simulink model "TrajectoryGenerator2DOF"  (R2023b)
settings: Solver=FixedStepDiscrete  StartTime=0.0  StopTime=1.538*1.4  FixedStep=0.002  RelTol=1e-3
undefined symbols (not defined in the file or in its folder): M_z, Smoothers, Ts
(part 2 of 3)

== system TrajectoryGenerator2DOF/Trajectory Generator10/M23 ==
  x : Inport
  Discrete FIR Filter1 : DiscreteFir  Coefficients=1/N/Ts*[1 zeros(1,N-1) -1]  InitialStates=Q0  SampleTime=Ts
  Discrete Filter : DiscreteFilter  Numerator=[0 Ts]  Denominator=[1 -1]  InitialStates=Q0  SampleTime=Ts
  y : Outport
  dy : Outport  Port=2
  wires:
  Discrete FIR Filter1/1 -> Discrete Filter/1, dy/1
  x/1 -> Discrete FIR Filter1/1
  Discrete Filter/1 -> y/1

== system TrajectoryGenerator2DOF/Trajectory Generator10/M24 ==
  x : Inport
  Discrete FIR Filter1 : DiscreteFir  Coefficients=1/N/Ts*[1 zeros(1,N-1) -1]  InitialStates=Q0  SampleTime=Ts
  Discrete Filter : DiscreteFilter  Numerator=[0 Ts]  Denominator=[1 -1]  InitialStates=Q0  SampleTime=Ts
  y : Outport
  dy : Outport  Port=2
  wires:
  Discrete FIR Filter1/1 -> Discrete Filter/1, dy/1
  x/1 -> Discrete FIR Filter1/1
  Discrete Filter/1 -> y/1

== system TrajectoryGenerator2DOF/Trajectory Generator10/M33 ==
  x : Inport
  Discrete FIR Filter1 : DiscreteFir  Coefficients=1/N/Ts*[1 zeros(1,N-1) -1]  InitialStates=Q0  SampleTime=Ts
  Discrete Filter : DiscreteFilter  Numerator=[0 Ts]  Denominator=[1 -1]  InitialStates=Q0  SampleTime=Ts
  y : Outport
  dy : Outport  Port=2
  wires:
  Discrete FIR Filter1/1 -> Discrete Filter/1, dy/1
  x/1 -> Discrete FIR Filter1/1
  Discrete Filter/1 -> y/1

== system TrajectoryGenerator2DOF/Trajectory Generator10/M34 ==
  x : Inport
  Discrete FIR Filter1 : DiscreteFir  Coefficients=1/N/Ts*[1 zeros(1,N-1) -1]  InitialStates=Q0  SampleTime=Ts
  Discrete Filter : DiscreteFilter  Numerator=[0 Ts]  Denominator=[1 -1]  InitialStates=Q0  SampleTime=Ts
  y : Outport
  dy : Outport  Port=2
  wires:
  Discrete FIR Filter1/1 -> Discrete Filter/1, dy/1
  x/1 -> Discrete FIR Filter1/1
  Discrete Filter/1 -> y/1

== system TrajectoryGenerator2DOF/Trajectory Generator10/M44 ==
  x : Inport
  Discrete FIR Filter1 : DiscreteFir  Coefficients=1/N/Ts*[1 zeros(1,N-1) -1]  InitialStates=Q0  SampleTime=Ts
  Discrete Filter : DiscreteFilter  Numerator=[0 Ts]  Denominator=[1 -1]  InitialStates=Q0  SampleTime=Ts
  y : Outport
  dy : Outport  Port=2
  wires:
  Discrete FIR Filter1/1 -> Discrete Filter/1, dy/1
  x/1 -> Discrete FIR Filter1/1
  Discrete Filter/1 -> y/1

== system TrajectoryGenerator2DOF/Trajectory Generator11/M11 ==
  x : Inport
  Discrete FIR Filter1 : DiscreteFir  Coefficients=1/N/Ts*[1 zeros(1,N-1) -1]  InitialStates=Q0  SampleTime=Ts
  Discrete Filter : DiscreteFilter  Numerator=[0 Ts]  Denominator=[1 -1]  InitialStates=Q0  SampleTime=Ts
  y : Outport
  dy : Outport  Port=2
  wires:
  Discrete FIR Filter1/1 -> Discrete Filter/1, dy/1
  x/1 -> Discrete FIR Filter1/1
  Discrete Filter/1 -> y/1

== system TrajectoryGenerator2DOF/Trajectory Generator11/M12 ==
  x : Inport
  Discrete FIR Filter1 : DiscreteFir  Coefficients=1/N/Ts*[1 zeros(1,N-1) -1]  InitialStates=Q0  SampleTime=Ts
  Discrete Filter : DiscreteFilter  Numerator=[0 Ts]  Denominator=[1 -1]  InitialStates=Q0  SampleTime=Ts
  y : Outport
  dy : Outport  Port=2
  wires:
  Discrete FIR Filter1/1 -> Discrete Filter/1, dy/1
  x/1 -> Discrete FIR Filter1/1
  Discrete Filter/1 -> y/1

== system TrajectoryGenerator2DOF/Trajectory Generator11/M13 ==
  x : Inport
  Discrete FIR Filter1 : DiscreteFir  Coefficients=1/N/Ts*[1 zeros(1,N-1) -1]  InitialStates=Q0  SampleTime=Ts
  Discrete Filter : DiscreteFilter  Numerator=[0 Ts]  Denominator=[1 -1]  InitialStates=Q0  SampleTime=Ts
  y : Outport
  dy : Outport  Port=2
  wires:
  Discrete FIR Filter1/1 -> Discrete Filter/1, dy/1
  x/1 -> Discrete FIR Filter1/1
  Discrete Filter/1 -> y/1

== system TrajectoryGenerator2DOF/Trajectory Generator11/M14 ==
  x : Inport
  Discrete FIR Filter1 : DiscreteFir  Coefficients=1/N/Ts*[1 zeros(1,N-1) -1]  InitialStates=Q0  SampleTime=Ts
  Discrete Filter : DiscreteFilter  Numerator=[0 Ts]  Denominator=[1 -1]  InitialStates=Q0  SampleTime=Ts
  y : Outport
  dy : Outport  Port=2
  wires:
  Discrete FIR Filter1/1 -> Discrete Filter/1, dy/1
  x/1 -> Discrete FIR Filter1/1
  Discrete Filter/1 -> y/1

== system TrajectoryGenerator2DOF/Trajectory Generator11/M22 ==
  x : Inport
  Discrete FIR Filter1 : DiscreteFir  Coefficients=1/N/Ts*[1 zeros(1,N-1) -1]  InitialStates=Q0  SampleTime=Ts
  Discrete Filter : DiscreteFilter  Numerator=[0 Ts]  Denominator=[1 -1]  InitialStates=Q0  SampleTime=Ts
  y : Outport
  dy : Outport  Port=2
  wires:
  Discrete FIR Filter1/1 -> Discrete Filter/1, dy/1
  x/1 -> Discrete FIR Filter1/1
  Discrete Filter/1 -> y/1

== system TrajectoryGenerator2DOF/Trajectory Generator11/M23 ==
  x : Inport
  Discrete FIR Filter1 : DiscreteFir  Coefficients=1/N/Ts*[1 zeros(1,N-1) -1]  InitialStates=Q0  SampleTime=Ts
  Discrete Filter : DiscreteFilter  Numerator=[0 Ts]  Denominator=[1 -1]  InitialStates=Q0  SampleTime=Ts
  y : Outport
  dy : Outport  Port=2
  wires:
  Discrete FIR Filter1/1 -> Discrete Filter/1, dy/1
  x/1 -> Discrete FIR Filter1/1
  Discrete Filter/1 -> y/1

== system TrajectoryGenerator2DOF/Trajectory Generator11/M24 ==
  x : Inport
  Discrete FIR Filter1 : DiscreteFir  Coefficients=1/N/Ts*[1 zeros(1,N-1) -1]  InitialStates=Q0  SampleTime=Ts
  Discrete Filter : DiscreteFilter  Numerator=[0 Ts]  Denominator=[1 -1]  InitialStates=Q0  SampleTime=Ts
  y : Outport
  dy : Outport  Port=2
  wires:
  Discrete FIR Filter1/1 -> Discrete Filter/1, dy/1
  x/1 -> Discrete FIR Filter1/1
  Discrete Filter/1 -> y/1

== system TrajectoryGenerator2DOF/Trajectory Generator11/M33 ==
  x : Inport
  Discrete FIR Filter1 : DiscreteFir  Coefficients=1/N/Ts*[1 zeros(1,N-1) -1]  InitialStates=Q0  SampleTime=Ts
  Discrete Filter : DiscreteFilter  Numerator=[0 Ts]  Denominator=[1 -1]  InitialStates=Q0  SampleTime=Ts
  y : Outport
  dy : Outport  Port=2
  wires:
  Discrete FIR Filter1/1 -> Discrete Filter/1, dy/1
  x/1 -> Discrete FIR Filter1/1
  Discrete Filter/1 -> y/1

== system TrajectoryGenerator2DOF/Trajectory Generator11/M34 ==
  x : Inport
  Discrete FIR Filter1 : DiscreteFir  Coefficients=1/N/Ts*[1 zeros(1,N-1) -1]  InitialStates=Q0  SampleTime=Ts
  Discrete Filter : DiscreteFilter  Numerator=[0 Ts]  Denominator=[1 -1]  InitialStates=Q0  SampleTime=Ts
  y : Outport
  dy : Outport  Port=2
  wires:
  Discrete FIR Filter1/1 -> Discrete Filter/1, dy/1
  x/1 -> Discrete FIR Filter1/1
  Discrete Filter/1 -> y/1

== system TrajectoryGenerator2DOF/Trajectory Generator11/M44 ==
  x : Inport
  Discrete FIR Filter1 : DiscreteFir  Coefficients=1/N/Ts*[1 zeros(1,N-1) -1]  InitialStates=Q0  SampleTime=Ts
  Discrete Filter : DiscreteFilter  Numerator=[0 Ts]  Denominator=[1 -1]  InitialStates=Q0  SampleTime=Ts
  y : Outport
  dy : Outport  Port=2
  wires:
  Discrete FIR Filter1/1 -> Discrete Filter/1, dy/1
  x/1 -> Discrete FIR Filter1/1
  Discrete Filter/1 -> y/1

== system TrajectoryGenerator2DOF/Trajectory Generator12/M11 ==
  x : Inport
  Discrete FIR Filter1 : DiscreteFir  Coefficients=1/N/Ts*[1 zeros(1,N-1) -1]  InitialStates=Q0  SampleTime=Ts
  Discrete Filter : DiscreteFilter  Numerator=[0 Ts]  Denominator=[1 -1]  InitialStates=Q0  SampleTime=Ts
  y : Outport
  dy : Outport  Port=2
  wires:
  Discrete FIR Filter1/1 -> Discrete Filter/1, dy/1
  x/1 -> Discrete FIR Filter1/1
  Discrete Filter/1 -> y/1

== system TrajectoryGenerator2DOF/Trajectory Generator12/M12 ==
  x : Inport
  Discrete FIR Filter1 : DiscreteFir  Coefficients=1/N/Ts*[1 zeros(1,N-1) -1]  InitialStates=Q0  SampleTime=Ts
  Discrete Filter : DiscreteFilter  Numerator=[0 Ts]  Denominator=[1 -1]  InitialStates=Q0  SampleTime=Ts
  y : Outport
  dy : Outport  Port=2
  wires:
  Discrete FIR Filter1/1 -> Discrete Filter/1, dy/1
  x/1 -> Discrete FIR Filter1/1
  Discrete Filter/1 -> y/1

== system TrajectoryGenerator2DOF/Trajectory Generator12/M13 ==
  x : Inport
  Discrete FIR Filter1 : DiscreteFir  Coefficients=1/N/Ts*[1 zeros(1,N-1) -1]  InitialStates=Q0  SampleTime=Ts
  Discrete Filter : DiscreteFilter  Numerator=[0 Ts]  Denominator=[1 -1]  InitialStates=Q0  SampleTime=Ts
  y : Outport
  dy : Outport  Port=2
  wires:
  Discrete FIR Filter1/1 -> Discrete Filter/1, dy/1
  x/1 -> Discrete FIR Filter1/1
  Discrete Filter/1 -> y/1

== system TrajectoryGenerator2DOF/Trajectory Generator12/M14 ==
  x : Inport
  Discrete FIR Filter1 : DiscreteFir  Coefficients=1/N/Ts*[1 zeros(1,N-1) -1]  InitialStates=Q0  SampleTime=Ts
  Discrete Filter : DiscreteFilter  Numerator=[0 Ts]  Denominator=[1 -1]  InitialStates=Q0  SampleTime=Ts
  y : Outport
  dy : Outport  Port=2
  wires:
  Discrete FIR Filter1/1 -> Discrete Filter/1, dy/1
  x/1 -> Discrete FIR Filter1/1
  Discrete Filter/1 -> y/1

== system TrajectoryGenerator2DOF/Trajectory Generator12/M22 ==
  x : Inport
  Discrete FIR Filter1 : DiscreteFir  Coefficients=1/N/Ts*[1 zeros(1,N-1) -1]  InitialStates=Q0  SampleTime=Ts
  Discrete Filter : DiscreteFilter  Numerator=[0 Ts]  Denominator=[1 -1]  InitialStates=Q0  SampleTime=Ts
  y : Outport
  dy : Outport  Port=2
  wires:
  Discrete FIR Filter1/1 -> Discrete Filter/1, dy/1
  x/1 -> Discrete FIR Filter1/1
  Discrete Filter/1 -> y/1

== system TrajectoryGenerator2DOF/Trajectory Generator12/M23 ==
  x : Inport
  Discrete FIR Filter1 : DiscreteFir  Coefficients=1/N/Ts*[1 zeros(1,N-1) -1]  InitialStates=Q0  SampleTime=Ts
  Discrete Filter : DiscreteFilter  Numerator=[0 Ts]  Denominator=[1 -1]  InitialStates=Q0  SampleTime=Ts
  y : Outport
  dy : Outport  Port=2
  wires:
  Discrete FIR Filter1/1 -> Discrete Filter/1, dy/1
  x/1 -> Discrete FIR Filter1/1
  Discrete Filter/1 -> y/1

== system TrajectoryGenerator2DOF/Trajectory Generator12/M24 ==
  x : Inport
  Discrete FIR Filter1 : DiscreteFir  Coefficients=1/N/Ts*[1 zeros(1,N-1) -1]  InitialStates=Q0  SampleTime=Ts
  Discrete Filter : DiscreteFilter  Numerator=[0 Ts]  Denominator=[1 -1]  InitialStates=Q0  SampleTime=Ts
  y : Outport
  dy : Outport  Port=2
  wires:
  Discrete FIR Filter1/1 -> Discrete Filter/1, dy/1
  x/1 -> Discrete FIR Filter1/1
  Discrete Filter/1 -> y/1

== system TrajectoryGenerator2DOF/Trajectory Generator12/M33 ==
  x : Inport
  Discrete FIR Filter1 : DiscreteFir  Coefficients=1/N/Ts*[1 zeros(1,N-1) -1]  InitialStates=Q0  SampleTime=Ts
  Discrete Filter : DiscreteFilter  Numerator=[0 Ts]  Denominator=[1 -1]  InitialStates=Q0  SampleTime=Ts
  y : Outport
  dy : Outport  Port=2
  wires:
  Discrete FIR Filter1/1 -> Discrete Filter/1, dy/1
  x/1 -> Discrete FIR Filter1/1
  Discrete Filter/1 -> y/1

== system TrajectoryGenerator2DOF/Trajectory Generator12/M34 ==
  x : Inport
  Discrete FIR Filter1 : DiscreteFir  Coefficients=1/N/Ts*[1 zeros(1,N-1) -1]  InitialStates=Q0  SampleTime=Ts
  Discrete Filter : DiscreteFilter  Numerator=[0 Ts]  Denominator=[1 -1]  InitialStates=Q0  SampleTime=Ts
  y : Outport
  dy : Outport  Port=2
  wires:
  Discrete FIR Filter1/1 -> Discrete Filter/1, dy/1
  x/1 -> Discrete FIR Filter1/1
  Discrete Filter/1 -> y/1

== system TrajectoryGenerator2DOF/Trajectory Generator12/M44 ==
  x : Inport
  Discrete FIR Filter1 : DiscreteFir  Coefficients=1/N/Ts*[1 zeros(1,N-1) -1]  InitialStates=Q0  SampleTime=Ts
  Discrete Filter : DiscreteFilter  Numerator=[0 Ts]  Denominator=[1 -1]  InitialStates=Q0  SampleTime=Ts
  y : Outport
  dy : Outport  Port=2
  wires:
  Discrete FIR Filter1/1 -> Discrete Filter/1, dy/1
  x/1 -> Discrete FIR Filter1/1
  Discrete Filter/1 -> y/1

== system TrajectoryGenerator2DOF/Trajectory Generator13/M11 ==
  x : Inport
  Discrete FIR Filter1 : DiscreteFir  Coefficients=1/N/Ts*[1 zeros(1,N-1) -1]  InitialStates=Q0  SampleTime=Ts
  Discrete Filter : DiscreteFilter  Numerator=[0 Ts]  Denominator=[1 -1]  InitialStates=Q0  SampleTime=Ts
  y : Outport
  dy : Outport  Port=2
  wires:
  Discrete FIR Filter1/1 -> Discrete Filter/1, dy/1
  x/1 -> Discrete FIR Filter1/1
  Discrete Filter/1 -> y/1

== system TrajectoryGenerator2DOF/Trajectory Generator13/M12 ==
  x : Inport
  Discrete FIR Filter1 : DiscreteFir  Coefficients=1/N/Ts*[1 zeros(1,N-1) -1]  InitialStates=Q0  SampleTime=Ts
  Discrete Filter : DiscreteFilter  Numerator=[0 Ts]  Denominator=[1 -1]  InitialStates=Q0  SampleTime=Ts
  y : Outport
  dy : Outport  Port=2
  wires:
  Discrete FIR Filter1/1 -> Discrete Filter/1, dy/1
  x/1 -> Discrete FIR Filter1/1
  Discrete Filter/1 -> y/1

== system TrajectoryGenerator2DOF/Trajectory Generator13/M13 ==
  x : Inport
  Discrete FIR Filter1 : DiscreteFir  Coefficients=1/N/Ts*[1 zeros(1,N-1) -1]  InitialStates=Q0  SampleTime=Ts
  Discrete Filter : DiscreteFilter  Numerator=[0 Ts]  Denominator=[1 -1]  InitialStates=Q0  SampleTime=Ts
  y : Outport
  dy : Outport  Port=2
  wires:
  Discrete FIR Filter1/1 -> Discrete Filter/1, dy/1
  x/1 -> Discrete FIR Filter1/1
  Discrete Filter/1 -> y/1

== system TrajectoryGenerator2DOF/Trajectory Generator13/M14 ==
  x : Inport
  Discrete FIR Filter1 : DiscreteFir  Coefficients=1/N/Ts*[1 zeros(1,N-1) -1]  InitialStates=Q0  SampleTime=Ts
  Discrete Filter : DiscreteFilter  Numerator=[0 Ts]  Denominator=[1 -1]  InitialStates=Q0  SampleTime=Ts
  y : Outport
  dy : Outport  Port=2
  wires:
  Discrete FIR Filter1/1 -> Discrete Filter/1, dy/1
  x/1 -> Discrete FIR Filter1/1
  Discrete Filter/1 -> y/1

== system TrajectoryGenerator2DOF/Trajectory Generator13/M22 ==
  x : Inport
  Discrete FIR Filter1 : DiscreteFir  Coefficients=1/N/Ts*[1 zeros(1,N-1) -1]  InitialStates=Q0  SampleTime=Ts
  Discrete Filter : DiscreteFilter  Numerator=[0 Ts]  Denominator=[1 -1]  InitialStates=Q0  SampleTime=Ts
  y : Outport
  dy : Outport  Port=2
  wires:
  Discrete FIR Filter1/1 -> Discrete Filter/1, dy/1
  x/1 -> Discrete FIR Filter1/1
  Discrete Filter/1 -> y/1

== system TrajectoryGenerator2DOF/Trajectory Generator13/M23 ==
  x : Inport
  Discrete FIR Filter1 : DiscreteFir  Coefficients=1/N/Ts*[1 zeros(1,N-1) -1]  InitialStates=Q0  SampleTime=Ts
  Discrete Filter : DiscreteFilter  Numerator=[0 Ts]  Denominator=[1 -1]  InitialStates=Q0  SampleTime=Ts
  y : Outport
  dy : Outport  Port=2
  wires:
  Discrete FIR Filter1/1 -> Discrete Filter/1, dy/1
  x/1 -> Discrete FIR Filter1/1
  Discrete Filter/1 -> y/1

== system TrajectoryGenerator2DOF/Trajectory Generator13/M24 ==
  x : Inport
  Discrete FIR Filter1 : DiscreteFir  Coefficients=1/N/Ts*[1 zeros(1,N-1) -1]  InitialStates=Q0  SampleTime=Ts
  Discrete Filter : DiscreteFilter  Numerator=[0 Ts]  Denominator=[1 -1]  InitialStates=Q0  SampleTime=Ts
  y : Outport
  dy : Outport  Port=2
  wires:
  Discrete FIR Filter1/1 -> Discrete Filter/1, dy/1
  x/1 -> Discrete FIR Filter1/1
  Discrete Filter/1 -> y/1

== system TrajectoryGenerator2DOF/Trajectory Generator13/M33 ==
  x : Inport
  Discrete FIR Filter1 : DiscreteFir  Coefficients=1/N/Ts*[1 zeros(1,N-1) -1]  InitialStates=Q0  SampleTime=Ts
  Discrete Filter : DiscreteFilter  Numerator=[0 Ts]  Denominator=[1 -1]  InitialStates=Q0  SampleTime=Ts
  y : Outport
  dy : Outport  Port=2
  wires:
  Discrete FIR Filter1/1 -> Discrete Filter/1, dy/1
  x/1 -> Discrete FIR Filter1/1
  Discrete Filter/1 -> y/1

== system TrajectoryGenerator2DOF/Trajectory Generator13/M34 ==
  x : Inport
  Discrete FIR Filter1 : DiscreteFir  Coefficients=1/N/Ts*[1 zeros(1,N-1) -1]  InitialStates=Q0  SampleTime=Ts
  Discrete Filter : DiscreteFilter  Numerator=[0 Ts]  Denominator=[1 -1]  InitialStates=Q0  SampleTime=Ts
  y : Outport
  dy : Outport  Port=2
  wires:
  Discrete FIR Filter1/1 -> Discrete Filter/1, dy/1
  x/1 -> Discrete FIR Filter1/1
  Discrete Filter/1 -> y/1

== system TrajectoryGenerator2DOF/Trajectory Generator13/M44 ==
  x : Inport
  Discrete FIR Filter1 : DiscreteFir  Coefficients=1/N/Ts*[1 zeros(1,N-1) -1]  InitialStates=Q0  SampleTime=Ts
  Discrete Filter : DiscreteFilter  Numerator=[0 Ts]  Denominator=[1 -1]  InitialStates=Q0  SampleTime=Ts
  y : Outport
  dy : Outport  Port=2
  wires:
  Discrete FIR Filter1/1 -> Discrete Filter/1, dy/1
  x/1 -> Discrete FIR Filter1/1
  Discrete Filter/1 -> y/1

== system TrajectoryGenerator2DOF/Trajectory Generator14/M11 ==
  x : Inport
  Discrete FIR Filter1 : DiscreteFir  Coefficients=1/N/Ts*[1 zeros(1,N-1) -1]  InitialStates=Q0  SampleTime=Ts
  Discrete Filter : DiscreteFilter  Numerator=[0 Ts]  Denominator=[1 -1]  InitialStates=Q0  SampleTime=Ts
  y : Outport
  dy : Outport  Port=2
  wires:
  Discrete FIR Filter1/1 -> Discrete Filter/1, dy/1
  x/1 -> Discrete FIR Filter1/1
  Discrete Filter/1 -> y/1

== system TrajectoryGenerator2DOF/Trajectory Generator14/M12 ==
  x : Inport
  Discrete FIR Filter1 : DiscreteFir  Coefficients=1/N/Ts*[1 zeros(1,N-1) -1]  InitialStates=Q0  SampleTime=Ts
  Discrete Filter : DiscreteFilter  Numerator=[0 Ts]  Denominator=[1 -1]  InitialStates=Q0  SampleTime=Ts
  y : Outport
  dy : Outport  Port=2
  wires:
  Discrete FIR Filter1/1 -> Discrete Filter/1, dy/1
  x/1 -> Discrete FIR Filter1/1
  Discrete Filter/1 -> y/1

== system TrajectoryGenerator2DOF/Trajectory Generator14/M13 ==
  x : Inport
  Discrete FIR Filter1 : DiscreteFir  Coefficients=1/N/Ts*[1 zeros(1,N-1) -1]  InitialStates=Q0  SampleTime=Ts
  Discrete Filter : DiscreteFilter  Numerator=[0 Ts]  Denominator=[1 -1]  InitialStates=Q0  SampleTime=Ts
  y : Outport
  dy : Outport  Port=2
  wires:
  Discrete FIR Filter1/1 -> Discrete Filter/1, dy/1
  x/1 -> Discrete FIR Filter1/1
  Discrete Filter/1 -> y/1

== system TrajectoryGenerator2DOF/Trajectory Generator14/M14 ==
  x : Inport
  Discrete FIR Filter1 : DiscreteFir  Coefficients=1/N/Ts*[1 zeros(1,N-1) -1]  InitialStates=Q0  SampleTime=Ts
  Discrete Filter : DiscreteFilter  Numerator=[0 Ts]  Denominator=[1 -1]  InitialStates=Q0  SampleTime=Ts
  y : Outport
  dy : Outport  Port=2
  wires:
  Discrete FIR Filter1/1 -> Discrete Filter/1, dy/1
  x/1 -> Discrete FIR Filter1/1
  Discrete Filter/1 -> y/1

== system TrajectoryGenerator2DOF/Trajectory Generator14/M22 ==
  x : Inport
  Discrete FIR Filter1 : DiscreteFir  Coefficients=1/N/Ts*[1 zeros(1,N-1) -1]  InitialStates=Q0  SampleTime=Ts
  Discrete Filter : DiscreteFilter  Numerator=[0 Ts]  Denominator=[1 -1]  InitialStates=Q0  SampleTime=Ts
  y : Outport
  dy : Outport  Port=2
  wires:
  Discrete FIR Filter1/1 -> Discrete Filter/1, dy/1
  x/1 -> Discrete FIR Filter1/1
  Discrete Filter/1 -> y/1

== system TrajectoryGenerator2DOF/Trajectory Generator14/M23 ==
  x : Inport
  Discrete FIR Filter1 : DiscreteFir  Coefficients=1/N/Ts*[1 zeros(1,N-1) -1]  InitialStates=Q0  SampleTime=Ts
  Discrete Filter : DiscreteFilter  Numerator=[0 Ts]  Denominator=[1 -1]  InitialStates=Q0  SampleTime=Ts
  y : Outport
  dy : Outport  Port=2
  wires:
  Discrete FIR Filter1/1 -> Discrete Filter/1, dy/1
  x/1 -> Discrete FIR Filter1/1
  Discrete Filter/1 -> y/1

== system TrajectoryGenerator2DOF/Trajectory Generator14/M24 ==
  x : Inport
  Discrete FIR Filter1 : DiscreteFir  Coefficients=1/N/Ts*[1 zeros(1,N-1) -1]  InitialStates=Q0  SampleTime=Ts
  Discrete Filter : DiscreteFilter  Numerator=[0 Ts]  Denominator=[1 -1]  InitialStates=Q0  SampleTime=Ts
  y : Outport
  dy : Outport  Port=2
  wires:
  Discrete FIR Filter1/1 -> Discrete Filter/1, dy/1
  x/1 -> Discrete FIR Filter1/1
  Discrete Filter/1 -> y/1

== system TrajectoryGenerator2DOF/Trajectory Generator14/M33 ==
  x : Inport
  Discrete FIR Filter1 : DiscreteFir  Coefficients=1/N/Ts*[1 zeros(1,N-1) -1]  InitialStates=Q0  SampleTime=Ts
  Discrete Filter : DiscreteFilter  Numerator=[0 Ts]  Denominator=[1 -1]  InitialStates=Q0  SampleTime=Ts
  y : Outport
  dy : Outport  Port=2
  wires:
  Discrete FIR Filter1/1 -> Discrete Filter/1, dy/1
  x/1 -> Discrete FIR Filter1/1
  Discrete Filter/1 -> y/1

== system TrajectoryGenerator2DOF/Trajectory Generator14/M34 ==
  x : Inport
  Discrete FIR Filter1 : DiscreteFir  Coefficients=1/N/Ts*[1 zeros(1,N-1) -1]  InitialStates=Q0  SampleTime=Ts
  Discrete Filter : DiscreteFilter  Numerator=[0 Ts]  Denominator=[1 -1]  InitialStates=Q0  SampleTime=Ts
  y : Outport
  dy : Outport  Port=2
  wires:
  Discrete FIR Filter1/1 -> Discrete Filter/1, dy/1
  x/1 -> Discrete FIR Filter1/1
  Discrete Filter/1 -> y/1

== system TrajectoryGenerator2DOF/Trajectory Generator14/M44 ==
  x : Inport
  Discrete FIR Filter1 : DiscreteFir  Coefficients=1/N/Ts*[1 zeros(1,N-1) -1]  InitialStates=Q0  SampleTime=Ts
  Discrete Filter : DiscreteFilter  Numerator=[0 Ts]  Denominator=[1 -1]  InitialStates=Q0  SampleTime=Ts
  y : Outport
  dy : Outport  Port=2
  wires:
  Discrete FIR Filter1/1 -> Discrete Filter/1, dy/1
  x/1 -> Discrete FIR Filter1/1
  Discrete Filter/1 -> y/1

== system TrajectoryGenerator2DOF/Trajectory Generator2/M11 ==
  x : Inport
  Discrete FIR Filter1 : DiscreteFir  Coefficients=1/N/Ts*[1 zeros(1,N-1) -1]  InitialStates=Q0  SampleTime=Ts
  Discrete Filter : DiscreteFilter  Numerator=[0 Ts]  Denominator=[1 -1]  InitialStates=Q0  SampleTime=Ts
  y : Outport
  dy : Outport  Port=2
  wires:
  Discrete FIR Filter1/1 -> Discrete Filter/1, dy/1
  x/1 -> Discrete FIR Filter1/1
  Discrete Filter/1 -> y/1

== system TrajectoryGenerator2DOF/Trajectory Generator2/M12 ==
  x : Inport
  Discrete FIR Filter1 : DiscreteFir  Coefficients=1/N/Ts*[1 zeros(1,N-1) -1]  InitialStates=Q0  SampleTime=Ts
  Discrete Filter : DiscreteFilter  Numerator=[0 Ts]  Denominator=[1 -1]  InitialStates=Q0  SampleTime=Ts
  y : Outport
  dy : Outport  Port=2
  wires:
  Discrete FIR Filter1/1 -> Discrete Filter/1, dy/1
  x/1 -> Discrete FIR Filter1/1
  Discrete Filter/1 -> y/1

== system TrajectoryGenerator2DOF/Trajectory Generator2/M13 ==
  x : Inport
  Discrete FIR Filter1 : DiscreteFir  Coefficients=1/N/Ts*[1 zeros(1,N-1) -1]  InitialStates=Q0  SampleTime=Ts
  Discrete Filter : DiscreteFilter  Numerator=[0 Ts]  Denominator=[1 -1]  InitialStates=Q0  SampleTime=Ts
  y : Outport
  dy : Outport  Port=2
  wires:
  Discrete FIR Filter1/1 -> Discrete Filter/1, dy/1
  x/1 -> Discrete FIR Filter1/1
  Discrete Filter/1 -> y/1

== system TrajectoryGenerator2DOF/Trajectory Generator2/M14 ==
  x : Inport
  Discrete FIR Filter1 : DiscreteFir  Coefficients=1/N/Ts*[1 zeros(1,N-1) -1]  InitialStates=Q0  SampleTime=Ts
  Discrete Filter : DiscreteFilter  Numerator=[0 Ts]  Denominator=[1 -1]  InitialStates=Q0  SampleTime=Ts
  y : Outport
  dy : Outport  Port=2
  wires:
  Discrete FIR Filter1/1 -> Discrete Filter/1, dy/1
  x/1 -> Discrete FIR Filter1/1
  Discrete Filter/1 -> y/1

== system TrajectoryGenerator2DOF/Trajectory Generator2/M22 ==
  x : Inport
  Discrete FIR Filter1 : DiscreteFir  Coefficients=1/N/Ts*[1 zeros(1,N-1) -1]  InitialStates=Q0  SampleTime=Ts
  Discrete Filter : DiscreteFilter  Numerator=[0 Ts]  Denominator=[1 -1]  InitialStates=Q0  SampleTime=Ts
  y : Outport
  dy : Outport  Port=2
  wires:
  Discrete FIR Filter1/1 -> Discrete Filter/1, dy/1
  x/1 -> Discrete FIR Filter1/1
  Discrete Filter/1 -> y/1

== system TrajectoryGenerator2DOF/Trajectory Generator2/M23 ==
  x : Inport
  Discrete FIR Filter1 : DiscreteFir  Coefficients=1/N/Ts*[1 zeros(1,N-1) -1]  InitialStates=Q0  SampleTime=Ts
  Discrete Filter : DiscreteFilter  Numerator=[0 Ts]  Denominator=[1 -1]  InitialStates=Q0  SampleTime=Ts
  y : Outport
  dy : Outport  Port=2
  wires:
  Discrete FIR Filter1/1 -> Discrete Filter/1, dy/1
  x/1 -> Discrete FIR Filter1/1
  Discrete Filter/1 -> y/1

== system TrajectoryGenerator2DOF/Trajectory Generator2/M24 ==
  x : Inport
  Discrete FIR Filter1 : DiscreteFir  Coefficients=1/N/Ts*[1 zeros(1,N-1) -1]  InitialStates=Q0  SampleTime=Ts
  Discrete Filter : DiscreteFilter  Numerator=[0 Ts]  Denominator=[1 -1]  InitialStates=Q0  SampleTime=Ts
  y : Outport
  dy : Outport  Port=2
  wires:
  Discrete FIR Filter1/1 -> Discrete Filter/1, dy/1
  x/1 -> Discrete FIR Filter1/1
  Discrete Filter/1 -> y/1

== system TrajectoryGenerator2DOF/Trajectory Generator2/M33 ==
  x : Inport
  Discrete FIR Filter1 : DiscreteFir  Coefficients=1/N/Ts*[1 zeros(1,N-1) -1]  InitialStates=Q0  SampleTime=Ts
  Discrete Filter : DiscreteFilter  Numerator=[0 Ts]  Denominator=[1 -1]  InitialStates=Q0  SampleTime=Ts
  y : Outport
  dy : Outport  Port=2
  wires:
  Discrete FIR Filter1/1 -> Discrete Filter/1, dy/1
  x/1 -> Discrete FIR Filter1/1
  Discrete Filter/1 -> y/1

== system TrajectoryGenerator2DOF/Trajectory Generator2/M34 ==
  x : Inport
  Discrete FIR Filter1 : DiscreteFir  Coefficients=1/N/Ts*[1 zeros(1,N-1) -1]  InitialStates=Q0  SampleTime=Ts
  Discrete Filter : DiscreteFilter  Numerator=[0 Ts]  Denominator=[1 -1]  InitialStates=Q0  SampleTime=Ts
  y : Outport
  dy : Outport  Port=2
  wires:
  Discrete FIR Filter1/1 -> Discrete Filter/1, dy/1
  x/1 -> Discrete FIR Filter1/1
  Discrete Filter/1 -> y/1

== system TrajectoryGenerator2DOF/Trajectory Generator2/M44 ==
  x : Inport
  Discrete FIR Filter1 : DiscreteFir  Coefficients=1/N/Ts*[1 zeros(1,N-1) -1]  InitialStates=Q0  SampleTime=Ts
  Discrete Filter : DiscreteFilter  Numerator=[0 Ts]  Denominator=[1 -1]  InitialStates=Q0  SampleTime=Ts
  y : Outport
  dy : Outport  Port=2
  wires:
  Discrete FIR Filter1/1 -> Discrete Filter/1, dy/1
  x/1 -> Discrete FIR Filter1/1
  Discrete Filter/1 -> y/1

== system TrajectoryGenerator2DOF/Trajectory Generator3/M11 ==
  x : Inport
  Discrete FIR Filter1 : DiscreteFir  Coefficients=1/N/Ts*[1 zeros(1,N-1) -1]  InitialStates=Q0  SampleTime=Ts
  Discrete Filter : DiscreteFilter  Numerator=[0 Ts]  Denominator=[1 -1]  InitialStates=Q0  SampleTime=Ts
  y : Outport
  dy : Outport  Port=2
  wires:
  Discrete FIR Filter1/1 -> Discrete Filter/1, dy/1
  x/1 -> Discrete FIR Filter1/1
  Discrete Filter/1 -> y/1

== system TrajectoryGenerator2DOF/Trajectory Generator3/M12 ==
  x : Inport
  Discrete FIR Filter1 : DiscreteFir  Coefficients=1/N/Ts*[1 zeros(1,N-1) -1]  InitialStates=Q0  SampleTime=Ts
  Discrete Filter : DiscreteFilter  Numerator=[0 Ts]  Denominator=[1 -1]  InitialStates=Q0  SampleTime=Ts
  y : Outport
  dy : Outport  Port=2
  wires:
  Discrete FIR Filter1/1 -> Discrete Filter/1, dy/1
  x/1 -> Discrete FIR Filter1/1
  Discrete Filter/1 -> y/1

== system TrajectoryGenerator2DOF/Trajectory Generator3/M13 ==
  x : Inport
  Discrete FIR Filter1 : DiscreteFir  Coefficients=1/N/Ts*[1 zeros(1,N-1) -1]  InitialStates=Q0  SampleTime=Ts
  Discrete Filter : DiscreteFilter  Numerator=[0 Ts]  Denominator=[1 -1]  InitialStates=Q0  SampleTime=Ts
  y : Outport
  dy : Outport  Port=2
  wires:
  Discrete FIR Filter1/1 -> Discrete Filter/1, dy/1
  x/1 -> Discrete FIR Filter1/1
  Discrete Filter/1 -> y/1

== system TrajectoryGenerator2DOF/Trajectory Generator3/M14 ==
  x : Inport
  Discrete FIR Filter1 : DiscreteFir  Coefficients=1/N/Ts*[1 zeros(1,N-1) -1]  InitialStates=Q0  SampleTime=Ts
  Discrete Filter : DiscreteFilter  Numerator=[0 Ts]  Denominator=[1 -1]  InitialStates=Q0  SampleTime=Ts
  y : Outport
  dy : Outport  Port=2
  wires:
  Discrete FIR Filter1/1 -> Discrete Filter/1, dy/1
  x/1 -> Discrete FIR Filter1/1
  Discrete Filter/1 -> y/1

== system TrajectoryGenerator2DOF/Trajectory Generator3/M22 ==
  x : Inport
  Discrete FIR Filter1 : DiscreteFir  Coefficients=1/N/Ts*[1 zeros(1,N-1) -1]  InitialStates=Q0  SampleTime=Ts
  Discrete Filter : DiscreteFilter  Numerator=[0 Ts]  Denominator=[1 -1]  InitialStates=Q0  SampleTime=Ts
  y : Outport
  dy : Outport  Port=2
  wires:
  Discrete FIR Filter1/1 -> Discrete Filter/1, dy/1
  x/1 -> Discrete FIR Filter1/1
  Discrete Filter/1 -> y/1

== system TrajectoryGenerator2DOF/Trajectory Generator3/M23 ==
  x : Inport
  Discrete FIR Filter1 : DiscreteFir  Coefficients=1/N/Ts*[1 zeros(1,N-1) -1]  InitialStates=Q0  SampleTime=Ts
  Discrete Filter : DiscreteFilter  Numerator=[0 Ts]  Denominator=[1 -1]  InitialStates=Q0  SampleTime=Ts
  y : Outport
  dy : Outport  Port=2
  wires:
  Discrete FIR Filter1/1 -> Discrete Filter/1, dy/1
  x/1 -> Discrete FIR Filter1/1
  Discrete Filter/1 -> y/1

== system TrajectoryGenerator2DOF/Trajectory Generator3/M24 ==
  x : Inport
  Discrete FIR Filter1 : DiscreteFir  Coefficients=1/N/Ts*[1 zeros(1,N-1) -1]  InitialStates=Q0  SampleTime=Ts
  Discrete Filter : DiscreteFilter  Numerator=[0 Ts]  Denominator=[1 -1]  InitialStates=Q0  SampleTime=Ts
  y : Outport
  dy : Outport  Port=2
  wires:
  Discrete FIR Filter1/1 -> Discrete Filter/1, dy/1
  x/1 -> Discrete FIR Filter1/1
  Discrete Filter/1 -> y/1

== system TrajectoryGenerator2DOF/Trajectory Generator3/M33 ==
  x : Inport
  Discrete FIR Filter1 : DiscreteFir  Coefficients=1/N/Ts*[1 zeros(1,N-1) -1]  InitialStates=Q0  SampleTime=Ts
  Discrete Filter : DiscreteFilter  Numerator=[0 Ts]  Denominator=[1 -1]  InitialStates=Q0  SampleTime=Ts
  y : Outport
  dy : Outport  Port=2
  wires:
  Discrete FIR Filter1/1 -> Discrete Filter/1, dy/1
  x/1 -> Discrete FIR Filter1/1
  Discrete Filter/1 -> y/1

== system TrajectoryGenerator2DOF/Trajectory Generator3/M34 ==
  x : Inport
  Discrete FIR Filter1 : DiscreteFir  Coefficients=1/N/Ts*[1 zeros(1,N-1) -1]  InitialStates=Q0  SampleTime=Ts
  Discrete Filter : DiscreteFilter  Numerator=[0 Ts]  Denominator=[1 -1]  InitialStates=Q0  SampleTime=Ts
  y : Outport
  dy : Outport  Port=2
  wires:
  Discrete FIR Filter1/1 -> Discrete Filter/1, dy/1
  x/1 -> Discrete FIR Filter1/1
  Discrete Filter/1 -> y/1

== system TrajectoryGenerator2DOF/Trajectory Generator3/M44 ==
  x : Inport
  Discrete FIR Filter1 : DiscreteFir  Coefficients=1/N/Ts*[1 zeros(1,N-1) -1]  InitialStates=Q0  SampleTime=Ts
  Discrete Filter : DiscreteFilter  Numerator=[0 Ts]  Denominator=[1 -1]  InitialStates=Q0  SampleTime=Ts
  y : Outport
  dy : Outport  Port=2
  wires:
  Discrete FIR Filter1/1 -> Discrete Filter/1, dy/1
  x/1 -> Discrete FIR Filter1/1
  Discrete Filter/1 -> y/1

== system TrajectoryGenerator2DOF/Trajectory Generator4/M11 ==
  x : Inport
  Discrete FIR Filter1 : DiscreteFir  Coefficients=1/N/Ts*[1 zeros(1,N-1) -1]  InitialStates=Q0  SampleTime=Ts
  Discrete Filter : DiscreteFilter  Numerator=[0 Ts]  Denominator=[1 -1]  InitialStates=Q0  SampleTime=Ts
  y : Outport
  dy : Outport  Port=2
  wires:
  Discrete FIR Filter1/1 -> Discrete Filter/1, dy/1
  x/1 -> Discrete FIR Filter1/1
  Discrete Filter/1 -> y/1

== system TrajectoryGenerator2DOF/Trajectory Generator4/M12 ==
  x : Inport
  Discrete FIR Filter1 : DiscreteFir  Coefficients=1/N/Ts*[1 zeros(1,N-1) -1]  InitialStates=Q0  SampleTime=Ts
  Discrete Filter : DiscreteFilter  Numerator=[0 Ts]  Denominator=[1 -1]  InitialStates=Q0  SampleTime=Ts
  y : Outport
  dy : Outport  Port=2
  wires:
  Discrete FIR Filter1/1 -> Discrete Filter/1, dy/1
  x/1 -> Discrete FIR Filter1/1
  Discrete Filter/1 -> y/1

== system TrajectoryGenerator2DOF/Trajectory Generator4/M13 ==
  x : Inport
  Discrete FIR Filter1 : DiscreteFir  Coefficients=1/N/Ts*[1 zeros(1,N-1) -1]  InitialStates=Q0  SampleTime=Ts
  Discrete Filter : DiscreteFilter  Numerator=[0 Ts]  Denominator=[1 -1]  InitialStates=Q0  SampleTime=Ts
  y : Outport
  dy : Outport  Port=2
  wires:
  Discrete FIR Filter1/1 -> Discrete Filter/1, dy/1
  x/1 -> Discrete FIR Filter1/1
  Discrete Filter/1 -> y/1

== system TrajectoryGenerator2DOF/Trajectory Generator4/M14 ==
  x : Inport
  Discrete FIR Filter1 : DiscreteFir  Coefficients=1/N/Ts*[1 zeros(1,N-1) -1]  InitialStates=Q0  SampleTime=Ts
  Discrete Filter : DiscreteFilter  Numerator=[0 Ts]  Denominator=[1 -1]  InitialStates=Q0  SampleTime=Ts
  y : Outport
  dy : Outport  Port=2
  wires:
  Discrete FIR Filter1/1 -> Discrete Filter/1, dy/1
  x/1 -> Discrete FIR Filter1/1
  Discrete Filter/1 -> y/1

== system TrajectoryGenerator2DOF/Trajectory Generator4/M22 ==
  x : Inport
  Discrete FIR Filter1 : DiscreteFir  Coefficients=1/N/Ts*[1 zeros(1,N-1) -1]  InitialStates=Q0  SampleTime=Ts
  Discrete Filter : DiscreteFilter  Numerator=[0 Ts]  Denominator=[1 -1]  InitialStates=Q0  SampleTime=Ts
  y : Outport
  dy : Outport  Port=2
  wires:
  Discrete FIR Filter1/1 -> Discrete Filter/1, dy/1
  x/1 -> Discrete FIR Filter1/1
  Discrete Filter/1 -> y/1

== system TrajectoryGenerator2DOF/Trajectory Generator4/M23 ==
  x : Inport
  Discrete FIR Filter1 : DiscreteFir  Coefficients=1/N/Ts*[1 zeros(1,N-1) -1]  InitialStates=Q0  SampleTime=Ts
  Discrete Filter : DiscreteFilter  Numerator=[0 Ts]  Denominator=[1 -1]  InitialStates=Q0  SampleTime=Ts
  y : Outport
  dy : Outport  Port=2
  wires:
  Discrete FIR Filter1/1 -> Discrete Filter/1, dy/1
  x/1 -> Discrete FIR Filter1/1
  Discrete Filter/1 -> y/1

== system TrajectoryGenerator2DOF/Trajectory Generator4/M24 ==
  x : Inport
  Discrete FIR Filter1 : DiscreteFir  Coefficients=1/N/Ts*[1 zeros(1,N-1) -1]  InitialStates=Q0  SampleTime=Ts
  Discrete Filter : DiscreteFilter  Numerator=[0 Ts]  Denominator=[1 -1]  InitialStates=Q0  SampleTime=Ts
  y : Outport
  dy : Outport  Port=2
  wires:
  Discrete FIR Filter1/1 -> Discrete Filter/1, dy/1
  x/1 -> Discrete FIR Filter1/1
  Discrete Filter/1 -> y/1

== system TrajectoryGenerator2DOF/Trajectory Generator4/M33 ==
  x : Inport
  Discrete FIR Filter1 : DiscreteFir  Coefficients=1/N/Ts*[1 zeros(1,N-1) -1]  InitialStates=Q0  SampleTime=Ts
  Discrete Filter : DiscreteFilter  Numerator=[0 Ts]  Denominator=[1 -1]  InitialStates=Q0  SampleTime=Ts
  y : Outport
  dy : Outport  Port=2
  wires:
  Discrete FIR Filter1/1 -> Discrete Filter/1, dy/1
  x/1 -> Discrete FIR Filter1/1
  Discrete Filter/1 -> y/1

== system TrajectoryGenerator2DOF/Trajectory Generator4/M34 ==
  x : Inport
  Discrete FIR Filter1 : DiscreteFir  Coefficients=1/N/Ts*[1 zeros(1,N-1) -1]  InitialStates=Q0  SampleTime=Ts
  Discrete Filter : DiscreteFilter  Numerator=[0 Ts]  Denominator=[1 -1]  InitialStates=Q0  SampleTime=Ts
  y : Outport
  dy : Outport  Port=2
  wires:
  Discrete FIR Filter1/1 -> Discrete Filter/1, dy/1
  x/1 -> Discrete FIR Filter1/1
  Discrete Filter/1 -> y/1

== system TrajectoryGenerator2DOF/Trajectory Generator4/M44 ==
  x : Inport
  Discrete FIR Filter1 : DiscreteFir  Coefficients=1/N/Ts*[1 zeros(1,N-1) -1]  InitialStates=Q0  SampleTime=Ts
  Discrete Filter : DiscreteFilter  Numerator=[0 Ts]  Denominator=[1 -1]  InitialStates=Q0  SampleTime=Ts
  y : Outport
  dy : Outport  Port=2
  wires:
  Discrete FIR Filter1/1 -> Discrete Filter/1, dy/1
  x/1 -> Discrete FIR Filter1/1
  Discrete Filter/1 -> y/1

== system TrajectoryGenerator2DOF/Trajectory Generator5/M11 ==
  x : Inport
  Discrete FIR Filter1 : DiscreteFir  Coefficients=1/N/Ts*[1 zeros(1,N-1) -1]  InitialStates=Q0  SampleTime=Ts
  Discrete Filter : DiscreteFilter  Numerator=[0 Ts]  Denominator=[1 -1]  InitialStates=Q0  SampleTime=Ts
  y : Outport
  dy : Outport  Port=2
  wires:
  Discrete FIR Filter1/1 -> Discrete Filter/1, dy/1
  x/1 -> Discrete FIR Filter1/1
  Discrete Filter/1 -> y/1

== system TrajectoryGenerator2DOF/Trajectory Generator5/M12 ==
  x : Inport
  Discrete FIR Filter1 : DiscreteFir  Coefficients=1/N/Ts*[1 zeros(1,N-1) -1]  InitialStates=Q0  SampleTime=Ts
  Discrete Filter : DiscreteFilter  Numerator=[0 Ts]  Denominator=[1 -1]  InitialStates=Q0  SampleTime=Ts
  y : Outport
  dy : Outport  Port=2
  wires:
  Discrete FIR Filter1/1 -> Discrete Filter/1, dy/1
  x/1 -> Discrete FIR Filter1/1
  Discrete Filter/1 -> y/1

== system TrajectoryGenerator2DOF/Trajectory Generator5/M13 ==
  x : Inport
  Discrete FIR Filter1 : DiscreteFir  Coefficients=1/N/Ts*[1 zeros(1,N-1) -1]  InitialStates=Q0  SampleTime=Ts
  Discrete Filter : DiscreteFilter  Numerator=[0 Ts]  Denominator=[1 -1]  InitialStates=Q0  SampleTime=Ts
  y : Outport
  dy : Outport  Port=2
  wires:
  Discrete FIR Filter1/1 -> Discrete Filter/1, dy/1
  x/1 -> Discrete FIR Filter1/1
  Discrete Filter/1 -> y/1

== system TrajectoryGenerator2DOF/Trajectory Generator5/M14 ==
  x : Inport
  Discrete FIR Filter1 : DiscreteFir  Coefficients=1/N/Ts*[1 zeros(1,N-1) -1]  InitialStates=Q0  SampleTime=Ts
  Discrete Filter : DiscreteFilter  Numerator=[0 Ts]  Denominator=[1 -1]  InitialStates=Q0  SampleTime=Ts
  y : Outport
  dy : Outport  Port=2
  wires:
  Discrete FIR Filter1/1 -> Discrete Filter/1, dy/1
  x/1 -> Discrete FIR Filter1/1
  Discrete Filter/1 -> y/1

== system TrajectoryGenerator2DOF/Trajectory Generator5/M22 ==
  x : Inport
  Discrete FIR Filter1 : DiscreteFir  Coefficients=1/N/Ts*[1 zeros(1,N-1) -1]  InitialStates=Q0  SampleTime=Ts
  Discrete Filter : DiscreteFilter  Numerator=[0 Ts]  Denominator=[1 -1]  InitialStates=Q0  SampleTime=Ts
  y : Outport
  dy : Outport  Port=2
  wires:
  Discrete FIR Filter1/1 -> Discrete Filter/1, dy/1
  x/1 -> Discrete FIR Filter1/1
  Discrete Filter/1 -> y/1

== system TrajectoryGenerator2DOF/Trajectory Generator5/M23 ==
  x : Inport
  Discrete FIR Filter1 : DiscreteFir  Coefficients=1/N/Ts*[1 zeros(1,N-1) -1]  InitialStates=Q0  SampleTime=Ts
  Discrete Filter : DiscreteFilter  Numerator=[0 Ts]  Denominator=[1 -1]  InitialStates=Q0  SampleTime=Ts
  y : Outport
  dy : Outport  Port=2
  wires:
  Discrete FIR Filter1/1 -> Discrete Filter/1, dy/1
  x/1 -> Discrete FIR Filter1/1
  Discrete Filter/1 -> y/1

== system TrajectoryGenerator2DOF/Trajectory Generator5/M24 ==
  x : Inport
  Discrete FIR Filter1 : DiscreteFir  Coefficients=1/N/Ts*[1 zeros(1,N-1) -1]  InitialStates=Q0  SampleTime=Ts
  Discrete Filter : DiscreteFilter  Numerator=[0 Ts]  Denominator=[1 -1]  InitialStates=Q0  SampleTime=Ts
  y : Outport
  dy : Outport  Port=2
  wires:
  Discrete FIR Filter1/1 -> Discrete Filter/1, dy/1
  x/1 -> Discrete FIR Filter1/1
  Discrete Filter/1 -> y/1

== system TrajectoryGenerator2DOF/Trajectory Generator5/M33 ==
  x : Inport
  Discrete FIR Filter1 : DiscreteFir  Coefficients=1/N/Ts*[1 zeros(1,N-1) -1]  InitialStates=Q0  SampleTime=Ts
  Discrete Filter : DiscreteFilter  Numerator=[0 Ts]  Denominator=[1 -1]  InitialStates=Q0  SampleTime=Ts
  y : Outport
  dy : Outport  Port=2
  wires:
  Discrete FIR Filter1/1 -> Discrete Filter/1, dy/1
  x/1 -> Discrete FIR Filter1/1
  Discrete Filter/1 -> y/1

== system TrajectoryGenerator2DOF/Trajectory Generator5/M34 ==
  x : Inport
  Discrete FIR Filter1 : DiscreteFir  Coefficients=1/N/Ts*[1 zeros(1,N-1) -1]  InitialStates=Q0  SampleTime=Ts
  Discrete Filter : DiscreteFilter  Numerator=[0 Ts]  Denominator=[1 -1]  InitialStates=Q0  SampleTime=Ts
  y : Outport
  dy : Outport  Port=2
  wires:
  Discrete FIR Filter1/1 -> Discrete Filter/1, dy/1
  x/1 -> Discrete FIR Filter1/1
  Discrete Filter/1 -> y/1

== system TrajectoryGenerator2DOF/Trajectory Generator5/M44 ==
  x : Inport
  Discrete FIR Filter1 : DiscreteFir  Coefficients=1/N/Ts*[1 zeros(1,N-1) -1]  InitialStates=Q0  SampleTime=Ts
  Discrete Filter : DiscreteFilter  Numerator=[0 Ts]  Denominator=[1 -1]  InitialStates=Q0  SampleTime=Ts
  y : Outport
  dy : Outport  Port=2
  wires:
  Discrete FIR Filter1/1 -> Discrete Filter/1, dy/1
  x/1 -> Discrete FIR Filter1/1
  Discrete Filter/1 -> y/1

== system TrajectoryGenerator2DOF/Trajectory Generator6/M11 ==
  x : Inport
  Discrete FIR Filter1 : DiscreteFir  Coefficients=1/N/Ts*[1 zeros(1,N-1) -1]  InitialStates=Q0  SampleTime=Ts
  Discrete Filter : DiscreteFilter  Numerator=[0 Ts]  Denominator=[1 -1]  InitialStates=Q0  SampleTime=Ts
  y : Outport
  dy : Outport  Port=2
  wires:
  Discrete FIR Filter1/1 -> Discrete Filter/1, dy/1
  x/1 -> Discrete FIR Filter1/1
  Discrete Filter/1 -> y/1

== system TrajectoryGenerator2DOF/Trajectory Generator6/M12 ==
  x : Inport
  Discrete FIR Filter1 : DiscreteFir  Coefficients=1/N/Ts*[1 zeros(1,N-1) -1]  InitialStates=Q0  SampleTime=Ts
  Discrete Filter : DiscreteFilter  Numerator=[0 Ts]  Denominator=[1 -1]  InitialStates=Q0  SampleTime=Ts
  y : Outport
  dy : Outport  Port=2
  wires:
  Discrete FIR Filter1/1 -> Discrete Filter/1, dy/1
  x/1 -> Discrete FIR Filter1/1
  Discrete Filter/1 -> y/1

== system TrajectoryGenerator2DOF/Trajectory Generator6/M13 ==
  x : Inport
  Discrete FIR Filter1 : DiscreteFir  Coefficients=1/N/Ts*[1 zeros(1,N-1) -1]  InitialStates=Q0  SampleTime=Ts
  Discrete Filter : DiscreteFilter  Numerator=[0 Ts]  Denominator=[1 -1]  InitialStates=Q0  SampleTime=Ts
  y : Outport
  dy : Outport  Port=2
  wires:
  Discrete FIR Filter1/1 -> Discrete Filter/1, dy/1
  x/1 -> Discrete FIR Filter1/1
  Discrete Filter/1 -> y/1

== system TrajectoryGenerator2DOF/Trajectory Generator6/M14 ==
  x : Inport
  Discrete FIR Filter1 : DiscreteFir  Coefficients=1/N/Ts*[1 zeros(1,N-1) -1]  InitialStates=Q0  SampleTime=Ts
  Discrete Filter : DiscreteFilter  Numerator=[0 Ts]  Denominator=[1 -1]  InitialStates=Q0  SampleTime=Ts
  y : Outport
  dy : Outport  Port=2
  wires:
  Discrete FIR Filter1/1 -> Discrete Filter/1, dy/1
  x/1 -> Discrete FIR Filter1/1
  Discrete Filter/1 -> y/1

== system TrajectoryGenerator2DOF/Trajectory Generator6/M22 ==
  x : Inport
  Discrete FIR Filter1 : DiscreteFir  Coefficients=1/N/Ts*[1 zeros(1,N-1) -1]  InitialStates=Q0  SampleTime=Ts
  Discrete Filter : DiscreteFilter  Numerator=[0 Ts]  Denominator=[1 -1]  InitialStates=Q0  SampleTime=Ts
  y : Outport
  dy : Outport  Port=2
  wires:
  Discrete FIR Filter1/1 -> Discrete Filter/1, dy/1
  x/1 -> Discrete FIR Filter1/1
  Discrete Filter/1 -> y/1

== system TrajectoryGenerator2DOF/Trajectory Generator6/M23 ==
  x : Inport
  Discrete FIR Filter1 : DiscreteFir  Coefficients=1/N/Ts*[1 zeros(1,N-1) -1]  InitialStates=Q0  SampleTime=Ts
  Discrete Filter : DiscreteFilter  Numerator=[0 Ts]  Denominator=[1 -1]  InitialStates=Q0  SampleTime=Ts
  y : Outport
  dy : Outport  Port=2
  wires:
  Discrete FIR Filter1/1 -> Discrete Filter/1, dy/1
  x/1 -> Discrete FIR Filter1/1
  Discrete Filter/1 -> y/1

== system TrajectoryGenerator2DOF/Trajectory Generator6/M24 ==
  x : Inport
  Discrete FIR Filter1 : DiscreteFir  Coefficients=1/N/Ts*[1 zeros(1,N-1) -1]  InitialStates=Q0  SampleTime=Ts
  Discrete Filter : DiscreteFilter  Numerator=[0 Ts]  Denominator=[1 -1]  InitialStates=Q0  SampleTime=Ts
  y : Outport
  dy : Outport  Port=2
  wires:
  Discrete FIR Filter1/1 -> Discrete Filter/1, dy/1
  x/1 -> Discrete FIR Filter1/1
  Discrete Filter/1 -> y/1

== system TrajectoryGenerator2DOF/Trajectory Generator6/M33 ==
  x : Inport
  Discrete FIR Filter1 : DiscreteFir  Coefficients=1/N/Ts*[1 zeros(1,N-1) -1]  InitialStates=Q0  SampleTime=Ts
  Discrete Filter : DiscreteFilter  Numerator=[0 Ts]  Denominator=[1 -1]  InitialStates=Q0  SampleTime=Ts
  y : Outport
  dy : Outport  Port=2
  wires:
  Discrete FIR Filter1/1 -> Discrete Filter/1, dy/1
  x/1 -> Discrete FIR Filter1/1
  Discrete Filter/1 -> y/1

== system TrajectoryGenerator2DOF/Trajectory Generator6/M34 ==
  x : Inport
  Discrete FIR Filter1 : DiscreteFir  Coefficients=1/N/Ts*[1 zeros(1,N-1) -1]  InitialStates=Q0  SampleTime=Ts
  Discrete Filter : DiscreteFilter  Numerator=[0 Ts]  Denominator=[1 -1]  InitialStates=Q0  SampleTime=Ts
  y : Outport
  dy : Outport  Port=2
  wires:
  Discrete FIR Filter1/1 -> Discrete Filter/1, dy/1
  x/1 -> Discrete FIR Filter1/1
  Discrete Filter/1 -> y/1

== system TrajectoryGenerator2DOF/Trajectory Generator6/M44 ==
  x : Inport
  Discrete FIR Filter1 : DiscreteFir  Coefficients=1/N/Ts*[1 zeros(1,N-1) -1]  InitialStates=Q0  SampleTime=Ts
  Discrete Filter : DiscreteFilter  Numerator=[0 Ts]  Denominator=[1 -1]  InitialStates=Q0  SampleTime=Ts
  y : Outport
  dy : Outport  Port=2
  wires:
  Discrete FIR Filter1/1 -> Discrete Filter/1, dy/1
  x/1 -> Discrete FIR Filter1/1
  Discrete Filter/1 -> y/1

== system TrajectoryGenerator2DOF/Trajectory Generator7/M11 ==
  x : Inport
  Discrete FIR Filter1 : DiscreteFir  Coefficients=1/N/Ts*[1 zeros(1,N-1) -1]  InitialStates=Q0  SampleTime=Ts
  Discrete Filter : DiscreteFilter  Numerator=[0 Ts]  Denominator=[1 -1]  InitialStates=Q0  SampleTime=Ts
  y : Outport
  dy : Outport  Port=2
  wires:
  Discrete FIR Filter1/1 -> Discrete Filter/1, dy/1
  x/1 -> Discrete FIR Filter1/1
  Discrete Filter/1 -> y/1

== system TrajectoryGenerator2DOF/Trajectory Generator7/M12 ==
  x : Inport
  Discrete FIR Filter1 : DiscreteFir  Coefficients=1/N/Ts*[1 zeros(1,N-1) -1]  InitialStates=Q0  SampleTime=Ts
  Discrete Filter : DiscreteFilter  Numerator=[0 Ts]  Denominator=[1 -1]  InitialStates=Q0  SampleTime=Ts
  y : Outport
  dy : Outport  Port=2
  wires:
  Discrete FIR Filter1/1 -> Discrete Filter/1, dy/1
  x/1 -> Discrete FIR Filter1/1
  Discrete Filter/1 -> y/1

== system TrajectoryGenerator2DOF/Trajectory Generator7/M13 ==
  x : Inport
  Discrete FIR Filter1 : DiscreteFir  Coefficients=1/N/Ts*[1 zeros(1,N-1) -1]  InitialStates=Q0  SampleTime=Ts
  Discrete Filter : DiscreteFilter  Numerator=[0 Ts]  Denominator=[1 -1]  InitialStates=Q0  SampleTime=Ts
  y : Outport
  dy : Outport  Port=2
  wires:
  Discrete FIR Filter1/1 -> Discrete Filter/1, dy/1
  x/1 -> Discrete FIR Filter1/1
  Discrete Filter/1 -> y/1

== system TrajectoryGenerator2DOF/Trajectory Generator7/M14 ==
  x : Inport
  Discrete FIR Filter1 : DiscreteFir  Coefficients=1/N/Ts*[1 zeros(1,N-1) -1]  InitialStates=Q0  SampleTime=Ts
  Discrete Filter : DiscreteFilter  Numerator=[0 Ts]  Denominator=[1 -1]  InitialStates=Q0  SampleTime=Ts
  y : Outport
  dy : Outport  Port=2
  wires:
  Discrete FIR Filter1/1 -> Discrete Filter/1, dy/1
  x/1 -> Discrete FIR Filter1/1
  Discrete Filter/1 -> y/1

== system TrajectoryGenerator2DOF/Trajectory Generator7/M22 ==
  x : Inport
  Discrete FIR Filter1 : DiscreteFir  Coefficients=1/N/Ts*[1 zeros(1,N-1) -1]  InitialStates=Q0  SampleTime=Ts
  Discrete Filter : DiscreteFilter  Numerator=[0 Ts]  Denominator=[1 -1]  InitialStates=Q0  SampleTime=Ts
  y : Outport
  dy : Outport  Port=2
  wires:
  Discrete FIR Filter1/1 -> Discrete Filter/1, dy/1
  x/1 -> Discrete FIR Filter1/1
  Discrete Filter/1 -> y/1

== system TrajectoryGenerator2DOF/Trajectory Generator7/M23 ==
  x : Inport
  Discrete FIR Filter1 : DiscreteFir  Coefficients=1/N/Ts*[1 zeros(1,N-1) -1]  InitialStates=Q0  SampleTime=Ts
  Discrete Filter : DiscreteFilter  Numerator=[0 Ts]  Denominator=[1 -1]  InitialStates=Q0  SampleTime=Ts
  y : Outport
  dy : Outport  Port=2
  wires:
  Discrete FIR Filter1/1 -> Discrete Filter/1, dy/1
  x/1 -> Discrete FIR Filter1/1
  Discrete Filter/1 -> y/1

== system TrajectoryGenerator2DOF/Trajectory Generator7/M24 ==
  x : Inport
  Discrete FIR Filter1 : DiscreteFir  Coefficients=1/N/Ts*[1 zeros(1,N-1) -1]  InitialStates=Q0  SampleTime=Ts
  Discrete Filter : DiscreteFilter  Numerator=[0 Ts]  Denominator=[1 -1]  InitialStates=Q0  SampleTime=Ts
  y : Outport
  dy : Outport  Port=2
  wires:
  Discrete FIR Filter1/1 -> Discrete Filter/1, dy/1
  x/1 -> Discrete FIR Filter1/1
  Discrete Filter/1 -> y/1

== system TrajectoryGenerator2DOF/Trajectory Generator7/M33 ==
  x : Inport
  Discrete FIR Filter1 : DiscreteFir  Coefficients=1/N/Ts*[1 zeros(1,N-1) -1]  InitialStates=Q0  SampleTime=Ts
  Discrete Filter : DiscreteFilter  Numerator=[0 Ts]  Denominator=[1 -1]  InitialStates=Q0  SampleTime=Ts
  y : Outport
  dy : Outport  Port=2
  wires:
  Discrete FIR Filter1/1 -> Discrete Filter/1, dy/1
  x/1 -> Discrete FIR Filter1/1
  Discrete Filter/1 -> y/1

== system TrajectoryGenerator2DOF/Trajectory Generator7/M34 ==
  x : Inport
  Discrete FIR Filter1 : DiscreteFir  Coefficients=1/N/Ts*[1 zeros(1,N-1) -1]  InitialStates=Q0  SampleTime=Ts
  Discrete Filter : DiscreteFilter  Numerator=[0 Ts]  Denominator=[1 -1]  InitialStates=Q0  SampleTime=Ts
  y : Outport
  dy : Outport  Port=2
  wires:
  Discrete FIR Filter1/1 -> Discrete Filter/1, dy/1
  x/1 -> Discrete FIR Filter1/1
  Discrete Filter/1 -> y/1

== system TrajectoryGenerator2DOF/Trajectory Generator7/M44 ==
  x : Inport
  Discrete FIR Filter1 : DiscreteFir  Coefficients=1/N/Ts*[1 zeros(1,N-1) -1]  InitialStates=Q0  SampleTime=Ts
  Discrete Filter : DiscreteFilter  Numerator=[0 Ts]  Denominator=[1 -1]  InitialStates=Q0  SampleTime=Ts
  y : Outport
  dy : Outport  Port=2
  wires:
  Discrete FIR Filter1/1 -> Discrete Filter/1, dy/1
  x/1 -> Discrete FIR Filter1/1
  Discrete Filter/1 -> y/1

== system TrajectoryGenerator2DOF/Trajectory Generator8/M11 ==
  x : Inport
  Discrete FIR Filter1 : DiscreteFir  Coefficients=1/N/Ts*[1 zeros(1,N-1) -1]  InitialStates=Q0  SampleTime=Ts
  Discrete Filter : DiscreteFilter  Numerator=[0 Ts]  Denominator=[1 -1]  InitialStates=Q0  SampleTime=Ts
  y : Outport
  dy : Outport  Port=2
  wires:
  Discrete FIR Filter1/1 -> Discrete Filter/1, dy/1
  x/1 -> Discrete FIR Filter1/1
  Discrete Filter/1 -> y/1

== system TrajectoryGenerator2DOF/Trajectory Generator8/M12 ==
  x : Inport
  Discrete FIR Filter1 : DiscreteFir  Coefficients=1/N/Ts*[1 zeros(1,N-1) -1]  InitialStates=Q0  SampleTime=Ts
  Discrete Filter : DiscreteFilter  Numerator=[0 Ts]  Denominator=[1 -1]  InitialStates=Q0  SampleTime=Ts
  y : Outport
  dy : Outport  Port=2
  wires:
  Discrete FIR Filter1/1 -> Discrete Filter/1, dy/1
  x/1 -> Discrete FIR Filter1/1
  Discrete Filter/1 -> y/1

== system TrajectoryGenerator2DOF/Trajectory Generator8/M13 ==
  x : Inport
  Discrete FIR Filter1 : DiscreteFir  Coefficients=1/N/Ts*[1 zeros(1,N-1) -1]  InitialStates=Q0  SampleTime=Ts
  Discrete Filter : DiscreteFilter  Numerator=[0 Ts]  Denominator=[1 -1]  InitialStates=Q0  SampleTime=Ts
  y : Outport
  dy : Outport  Port=2
  wires:
  Discrete FIR Filter1/1 -> Discrete Filter/1, dy/1
  x/1 -> Discrete FIR Filter1/1
  Discrete Filter/1 -> y/1

== system TrajectoryGenerator2DOF/Trajectory Generator8/M14 ==
  x : Inport
  Discrete FIR Filter1 : DiscreteFir  Coefficients=1/N/Ts*[1 zeros(1,N-1) -1]  InitialStates=Q0  SampleTime=Ts
  Discrete Filter : DiscreteFilter  Numerator=[0 Ts]  Denominator=[1 -1]  InitialStates=Q0  SampleTime=Ts
  y : Outport
  dy : Outport  Port=2
  wires:
  Discrete FIR Filter1/1 -> Discrete Filter/1, dy/1
  x/1 -> Discrete FIR Filter1/1
  Discrete Filter/1 -> y/1

== system TrajectoryGenerator2DOF/Trajectory Generator8/M22 ==
  x : Inport
  Discrete FIR Filter1 : DiscreteFir  Coefficients=1/N/Ts*[1 zeros(1,N-1) -1]  InitialStates=Q0  SampleTime=Ts
  Discrete Filter : DiscreteFilter  Numerator=[0 Ts]  Denominator=[1 -1]  InitialStates=Q0  SampleTime=Ts
  y : Outport
  dy : Outport  Port=2
  wires:
  Discrete FIR Filter1/1 -> Discrete Filter/1, dy/1
  x/1 -> Discrete FIR Filter1/1
  Discrete Filter/1 -> y/1
